simulink model "LCK_AVP"  (R2018b)
settings: Solver=FixedStepDiscrete  StartTime=0.0  StopTime=inf  FixedStep=0.01  RelTol=1e-3
PreLoadFcn:
  | if exist('tl_preloadfcn','file'), tl_preloadfcn(gcs,'4.4.0.41'); end
PostLoadFcn:
  | if any(exist('dsrtsu_mdlpostloadfcn', 'file') ~= 0), dsrtsu_mdlpostloadfcn('Execute', bdroot); end
  | if exist('tl_postloadfcn','file'), tl_postloadfcn(gcs,'4.4.0.41'); end
InitFcn:
  | if exist('tlds_init','file'), tlds_init(gcs); end
StartFcn:
  | if exist('tlds_start','file'), tlds_start(gcs); end
StopFcn:
  | if exist('tlds_stop','file'), tlds_stop(gcs); end
values from neighbouring files (symbols this model uses):
  C_DEG2RAD = 0.0175    [LCK_Macro.sldd]
  C_KPH2MPS = 0.2778    [LCK_Macro.sldd]
  C_NEARZERO = 0.0001    [LCK_Macro.sldd]
  C_ONE = 1.0    [LCK_Macro.sldd]
  C_RAD2DEG = 57.2958    [LCK_Macro.sldd]
  C_ZERO = 0.0    [LCK_Macro.sldd]
  k_accel_pedal_pos_per_speed_x : value not decoded    [LCK_LogicPara.sldd]
  k_accel_pedal_pos_per_speed_z : value not decoded    [LCK_LogicPara.sldd]
  k_brake_suprress_hold = 1000.0    [LCK_LogicPara.sldd]
  k_driver_appl_torque_filt = 50.0    [LCK_LogicPara.sldd]
  k_driver_suppression_hold_time = 3000.0    [LCK_LogicPara.sldd]
  k_hands_on_wheel_hold_msec = 500.0    [LCK_LogicPara.sldd]
  k_hands_on_wheel_torque_hi = 0.2    [LCK_LogicPara.sldd]
  k_hands_on_wheel_torque_lo = 0.15    [LCK_LogicPara.sldd]
  k_handsoff_delay_cycles = 50.0    [LCK_LogicPara.sldd]
  k_handsoff_torq_Lo_CR = 0.3    [LCK_LogicPara.sldd]
  k_handson_delay_cycles = 5.0    [LCK_LogicPara.sldd]
  k_HighAccel_suppress_hold = 3000.0    [LCK_LogicPara.sldd]
  k_HLR_suprress_hold = 3000.0    [LCK_LogicPara.sldd]
  k_hs_StrAng_CR_threshold_z : value not decoded    [LCK_LogicPara.sldd]
  k_LC_Exit_Switch = 0.0    [LCK_LogicPara.sldd]
  k_LCG_Configured = 1.0    [LCK_LogicPara.sldd]
  k_LCK_A0_Rdy2Act_UseConst = 0.0    [LCK_LogicPara.sldd]
  k_LCK_A0Fac_ActSta : value not decoded    [LCK_CtrlPara.sldd]
  k_LCK_A0Fac_DrvStm : value not decoded    [LCK_CtrlPara.sldd]
  k_LCK_A0Shift_LftCurv : value not decoded    [LCK_CtrlPara.sldd]
  k_LCK_A0Shift_RgtCurv : value not decoded    [LCK_CtrlPara.sldd]
  k_LCK_A0Shift_StraLan = 0.0    [LCK_CtrlPara.sldd]
  k_LCK_A0ShiftFac_Dy_LftCurv : value not decoded    [LCK_CtrlPara.sldd]
  k_LCK_A0ShiftFac_Dy_RgtCurv : value not decoded    [LCK_CtrlPara.sldd]
  k_LCK_A0ShiftFac_Vspd : value not decoded    [LCK_CtrlPara.sldd]
  k_LCK_accel_inhibit_thold = 35.0    [LCK_LogicPara.sldd]
  k_LCK_Active2Ready_Mask = 255.0    [LCK_LogicPara.sldd]
  k_LCK_CvatRateBks : value not decoded    [LCK_CtrlPara.sldd]
  k_LCK_CvatrBks : value not decoded    [LCK_CtrlPara.sldd]
  k_LCK_DFac_Dy : value not decoded    [LCK_CtrlPara.sldd]
  k_LCK_DFac_Dy_Curv : value not decoded    [LCK_CtrlPara.sldd]
  k_LCK_DFac_HaCurCen : value not decoded    [LCK_CtrlPara.sldd]
  k_LCK_DFac_HaCurSid : value not decoded    [LCK_CtrlPara.sldd]
  k_LCK_DFac_HadCurCen : value not decoded    [LCK_CtrlPara.sldd]
  k_LCK_DFac_HadCurSid : value not decoded    [LCK_CtrlPara.sldd]
  k_LCK_DFac_HadStrCen : value not decoded    [LCK_CtrlPara.sldd]
  k_LCK_DFac_HadStrSid : value not decoded    [LCK_CtrlPara.sldd]
  k_LCK_DFac_HaStrCen : value not decoded    [LCK_CtrlPara.sldd]
  k_LCK_DFac_HaStrSid : value not decoded    [LCK_CtrlPara.sldd]
  k_LCK_DFac_Rad : value not decoded    [LCK_CtrlPara.sldd]
  k_LCK_DFac_SA_CurCen : value not decoded    [LCK_CtrlPara.sldd]
  k_LCK_DFac_SA_CurSid : value not decoded    [LCK_CtrlPara.sldd]
  k_LCK_DFac_SA_StrCen : value not decoded    [LCK_CtrlPara.sldd]
  k_LCK_DFac_SA_StrSid : value not decoded    [LCK_CtrlPara.sldd]
  k_LCK_DFac_SS_CurCen : value not decoded    [LCK_CtrlPara.sldd]
  k_LCK_DFac_SS_CurSid : value not decoded    [LCK_CtrlPara.sldd]
  k_LCK_DFac_SS_StrCen : value not decoded    [LCK_CtrlPara.sldd]
  k_LCK_DFac_SS_StrSid : value not decoded    [LCK_CtrlPara.sldd]
  k_LCK_DFac_Vspd : value not decoded    [LCK_CtrlPara.sldd]
  k_LCK_DlyTm_DrvStim = 0.2    [LCK_CtrlPara.sldd]
  k_LCK_DTermMax = 2.0    [LCK_CtrlPara.sldd]
  k_LCK_DyBks_Curv : value not decoded    [LCK_CtrlPara.sldd]
  k_LCK_Enable_POOnly = 1.0    [LCK_LogicPara.sldd]
  k_LCK_Entry_DistBuffer = 0.1    [LCK_LogicPara.sldd]
  k_LCK_Fac_Vspd2RngThr_FalRec = 0.23    [LCK_CtrlPara.sldd]
  k_LCK_Ffw_CvatSwh = 0.0    [LCK_CtrlPara.sldd]
  k_LCK_Ffw_DyBks : value not decoded    [LCK_CtrlPara.sldd]
  k_LCK_Ffw_TimCon_CmdFlt = 0.0    [LCK_CtrlPara.sldd]
  k_LCK_FfwDeltaFac_Rad_Lft : value not decoded    [LCK_CtrlPara.sldd]
  k_LCK_FfwDeltaFac_Rad_Rgt : value not decoded    [LCK_CtrlPara.sldd]
  k_LCK_FfwDeltaFac_Vspd : value not decoded    [LCK_CtrlPara.sldd]
  k_LCK_FfwFac_CvatRate_Lft : value not decoded    [LCK_CtrlPara.sldd]
  k_LCK_FfwFac_CvatRate_Rgt : value not decoded    [LCK_CtrlPara.sldd]
  k_LCK_FfwFac_Dy : value not decoded    [LCK_CtrlPara.sldd]
  k_LCK_FfwFac_Rad_Lft : value not decoded    [LCK_CtrlPara.sldd]
  k_LCK_FfwFac_Rad_Rgt : value not decoded    [LCK_CtrlPara.sldd]
  k_LCK_FfwFac_Vspd : value not decoded    [LCK_CtrlPara.sldd]
  k_LCK_FfwTorq_Cvat : value not decoded    [LCK_CtrlPara.sldd]
  k_LCK_HAFac_ActSta : value not decoded    [LCK_CtrlPara.sldd]
  k_LCK_HAFac_DrvStm : value not decoded    [LCK_CtrlPara.sldd]
  k_LCK_HaloTime = 2000.0    [LCK_LogicPara.sldd]
  k_LCK_HaloTime_Switch = 0.0    [LCK_LogicPara.sldd]
  k_LCK_HARFac_ActSta : value not decoded    [LCK_CtrlPara.sldd]
  k_LCK_HARFac_DrvStm : value not decoded    [LCK_CtrlPara.sldd]
  k_LCK_Hed_DyBks : value not decoded    [LCK_CtrlPara.sldd]
  k_LCK_HedAngDiffX : value not decoded    [LCK_CtrlPara.sldd]
  k_LCK_HedAngRateDiffX : value not decoded    [LCK_CtrlPara.sldd]
  k_LCK_HndsOnWhel_DlyTm_Idl2Rdy = 0.0    [LCK_LogicPara.sldd]
  k_LCK_host_veh_width = 1.86    [LCK_LogicPara.sldd]
  k_LCK_Idle2Ready_Mask = 239.0    [LCK_LogicPara.sldd]
  k_LCK_Junc_SusTime = 1.0    [LCK_LogicPara.sldd]
  k_LCK_KpKdDecSlopeLmt = 10.0    [LCK_CtrlPara.sldd]
  k_LCK_KpKdIncSlopeLmt = 5.0    [LCK_CtrlPara.sldd]
  k_LCK_Lat_Ctrl_DFac_Lft = 1.0    [LCK_CtrlPara.sldd]
  k_LCK_Lat_Ctrl_DFac_Rgt = 1.05    [LCK_CtrlPara.sldd]
  k_LCK_Lat_Ctrl_Kd = 0.8    [LCK_CtrlPara.sldd]
  k_LCK_Lat_Ctrl_Ki = 0.5    [LCK_CtrlPara.sldd]
  k_LCK_Lat_Ctrl_Kp = 0.7    [LCK_CtrlPara.sldd]
  k_LCK_Lat_Ctrl_Kp_NearGain = 0.7    [LCK_CtrlPara.sldd]
  k_LCK_Lat_Ctrl_PFac_Lft = 1.0    [LCK_CtrlPara.sldd]
  k_LCK_Lat_Ctrl_PFac_Rgt = 1.05    [LCK_CtrlPara.sldd]
  k_LCK_Lat_Ctrl_TimCon_CmdFlt = 5.0    [LCK_CtrlPara.sldd]
  k_LCK_Lat_DFac_Rad : value not decoded    [LCK_CtrlPara.sldd]
  k_LCK_Lat_DFac_SS_Cur : value not decoded    [LCK_CtrlPara.sldd]
  k_LCK_Lat_DFac_SS_Str : value not decoded    [LCK_CtrlPara.sldd]
  k_LCK_Lat_DFac_Vspd : value not decoded    [LCK_CtrlPara.sldd]
  k_LCK_Lat_DyBks : value not decoded    [LCK_CtrlPara.sldd]
  k_LCK_Lat_IFac_Rad : value not decoded    [LCK_CtrlPara.sldd]
  k_LCK_Lat_IFac_Vspd : value not decoded    [LCK_CtrlPara.sldd]
  k_LCK_Lat_ILmtFac_Dy_CurvLan : value not decoded    [LCK_CtrlPara.sldd]
  k_LCK_Lat_ILmtFac_Dy_StraLan : value not decoded    [LCK_CtrlPara.sldd]
  k_LCK_Lat_ILmtFac_Rad : value not decoded    [LCK_CtrlPara.sldd]
  k_LCK_Lat_ILmtFac_Rad_NearGain = 1.0    [LCK_CtrlPara.sldd]
  k_LCK_Lat_ILmtFac_Vspd_CurvLan : value not decoded    [LCK_CtrlPara.sldd]
  k_LCK_Lat_ILmtFac_Vspd_StraLan : value not decoded    [LCK_CtrlPara.sldd]
  k_LCK_Lat_ITermLmt_Dy = 1.0    [LCK_CtrlPara.sldd]
  k_LCK_Lat_KpKdDecSlopeLmt = 10.0    [LCK_CtrlPara.sldd]
  k_LCK_Lat_KpKdIncSlopeLmt = 10.0    [LCK_CtrlPara.sldd]
  k_LCK_Lat_PFac_Dy_InnLftCur : value not decoded    [LCK_CtrlPara.sldd]
  k_LCK_Lat_PFac_Dy_InnRgtCur : value not decoded    [LCK_CtrlPara.sldd]
  k_LCK_Lat_PFac_Dy_OutLftCur : value not decoded    [LCK_CtrlPara.sldd]
  k_LCK_Lat_PFac_Dy_OutRgtCur : value not decoded    [LCK_CtrlPara.sldd]
  k_LCK_Lat_PFac_Dy_Str : value not decoded    [LCK_CtrlPara.sldd]
  k_LCK_Lat_PFac_Rad : value not decoded    [LCK_CtrlPara.sldd]
  ... (+153 more)
undefined symbols (not defined in the file or in its folder): k_LCK_CurvBks, K_LCK_SPA0A1A2_LMRngCmp_y
libraries: LateralControl_fcns_lib x58, simulink x24
(part 11 of 48)

== system LCK_AVP/Lateral_Control_Module/Adas_Lateral_Control_LCK_Core/Module 9 ==
  Vspd : Inport
  Dy_0 : Inport  Port=2
  Hed_Ang : Inport  Port=3
  Hed_Ang_Rat : Inport  Port=4
  Steer_Ang : Inport  Port=5
  Steer_Spd : Inport  Port=6
  Road_Radius : Inport  Port=7
  Str_Flag : Inport  Port=8
  Cen_Flag : Inport  Port=9
  Bus Creator : BusCreator  Inputs=5
  Module 0 : Subsystem
  Module 1 : Subsystem
  LatCtrl_Info : Outport
  wires:
  Dy_0/1 -> Module 0/3(Dy_0)
  Hed_Ang/1 -> Module 0/1(Hed_Ang), Module 1/1(Hed_Ang)
  Str_Flag/1 -> Module 0/4(Str_Flag)
  Vspd/1 -> Module 0/5(Vspd)
  Road_Radius/1 -> Module 0/6(Road_Radius)
  Steer_Spd/1 -> Module 0/8(Steer_Spd)
  Hed_Ang_Rat/1 -> Module 1/2(Hed_Ang_Rat), Module 0/2(Hed_Ang_Diff_Rat)
  Module 1/1(LatCtrl_Cmd) -> Bus Creator/1  "LatCtrl_Cmd"
  Cen_Flag/1 -> Module 0/9(Cen_Flag)
  Bus Creator/1 -> LatCtrl_Info/1
  Steer_Ang/1 -> Module 0/7(Steer_Ang)
  Module 0/1(P_Gain) -> Bus Creator/4, Module 1/3(P_Gain)  "LatCtrl_P"
  Module 0/2(D_Gain) -> Bus Creator/5, Module 1/4(D_Gain)  "LatCtrl_D"
  Module 1/2(LatCtrl_P_Term) -> Bus Creator/2  "LatCtrl_PTerm"
  Module 1/3(LatCtrl_D_Term) -> Bus Creator/3  "LatCtrl_DTerm"

== system LCK_AVP/Lateral_Control_Module/Adas_Lateral_Control_LCK_Core/Process of SPP False Recognition ==
  LatCtrl_LCK_LanSigInputs : Inport
  LatCtrl_LCK_TrackSigInputs : Inport  Description=_GWMAB30P4.LCK.000_220_  Port=2
  Vspd : Inport  Port=3
  Bus Selector20 : BusSelector  OutputSignals=CIPV1ObjRange,CIPV1ObjTrackID
  Bus Selector21 : BusSelector  OutputSignals=VID_Lin_01_Range,VID_Lin_02_Range
  Constant10 : Constant  Value=0  OutDataTypeStr=uint8
  Constant2 : Constant  Value=4  OutDataTypeStr=uint8
  Constant5 : Constant  Value=0  OutDataTypeStr=uint8
  Constant6 : Constant  Value=2  OutDataTypeStr=uint8
  Constant8 : Constant  Value=2  OutDataTypeStr=uint8
  Constant9 : Constant  Value=3  OutDataTypeStr=uint8
  Divide1 : Product  Description=_GWMAB30P3.LCK.000_157_  Inputs=*/  OutDataTypeStr=single
  Product6 : Product
  Relational Operator : RelationalOperator  OutDataTypeStr=boolean  RndMeth=Nearest
  Relational Operator1 : RelationalOperator  Operator=>  OutDataTypeStr=boolean  RndMeth=Nearest
  Relational Operator2 : RelationalOperator  Operator=<  OutDataTypeStr=boolean  RndMeth=Nearest
  Sum3 : Sum  Description=_GWMAB30P2.LCK.000_1362_
  Switch1 : Switch  Description=_GWMAB30P2.LCK.000_1368_  Threshold=0.5  OutDataTypeStr=uint8
  Switch10 : Switch  Description=_GWMAB30P2.LCK.000_1368_  Threshold=0.5
  Switch8 : Switch  Description=_GWMAB30P2.LCK.000_1368_  Threshold=0.5  OutDataTypeStr=uint8
  k_LCK_Fac_Vspd2RngThr_FalRec : Constant  Value=k_LCK_Fac_Vspd2RngThr_FalRec
  k_LCK_RngThr_FalRec : Lookup_n-D  NumberOfTableDimensions=1  BreakpointsForDimension1=k_LCK_VspdBks  Table=k_LCK_RngThr_FalRec  ExtrapMethod=Clip  InternalRulePriority=Speed  RndMeth=Simplest  InputSameDT=on
  SPP_Recognition_Type : Outport
  wires:
  LatCtrl_LCK_LanSigInputs/1 -> Bus Selector21/1
  LatCtrl_LCK_TrackSigInputs/1 -> Bus Selector20/1
  Constant5/1 -> Relational Operator1/2
  Relational Operator2/1 -> Switch10/2
  k_LCK_Fac_Vspd2RngThr_FalRec/1 -> Product6/1
  Constant9/1 -> Switch10/3
  Constant10/1 -> Switch8/3
  Switch8/1 -> SPP_Recognition_Type/1
  Constant6/1 -> Divide1/2
  Constant8/1 -> Switch10/1
  Relational Operator/1 -> Switch8/2
  Relational Operator1/1 -> Switch1/2
  Constant2/1 -> Switch1/3
  Switch10/1 -> Switch1/1
  Switch1/1 -> Switch8/1
  Bus Selector20/2 -> Relational Operator1/1  "<CIPV1ObjTrackID>"
  Product6/1 -> Relational Operator2/1
  Bus Selector20/1 -> Relational Operator2/2  "<CIPV1ObjRange>"
  Vspd/1 -> Product6/2, k_LCK_RngThr_FalRec/1
  k_LCK_RngThr_FalRec/1 -> Relational Operator/1
  Bus Selector21/1 -> Sum3/1  "<VID_Lin_01_Range>"
  Bus Selector21/2 -> Sum3/2  "<VID_Lin_02_Range>"
  Sum3/1 -> Divide1/1
  Divide1/1 -> Relational Operator/2

== system LCK_AVP/Lateral_Control_Module/LCK_State_Ctrl/Det_Driver_Operation ==
  veh_speed_kph : Inport  Description=_GWMAB30P4.LCK.000_82_
  TorsionBarTorque : Inport  Description=_GWMH9P3.Latctrl.000_23_  Port=2
  Steer_Angle_iso : Inport  Description=_GWMH9P3.Latctrl.000_23_  Port=3
  BrkPedalApp : Inport  Description=_GWMH9P3.Latctrl.000_23_  Port=4
  AccPedalPosition : Inport  Description=_GWMH9P3.Latctrl.000_23_  Port=5
  Gear_Pos : Inport  Description=_GWMH9P3.Latctrl.000_23_  Port=6
  steer_angle_CR_iso : Inport  Description=_GWMH9P3.Latctrl.000_23_  Port=7
  DirectionIndSwitchPos : Inport  Description=_GACA26P3.Latctrl.000_20_  Port=8
  LCK_Mode : Inport  Port=9
  Final_Torq_Cmd : Inport  Port=10
  Det_Driver_Steer_Override : Subsystem  Description=_GWMAB30P4.Latctrl.000_122_  TreatAsAtomicUnit=on
  Det_Driver_Suppression : Subsystem
  Det_Hands_on_Wheel : Subsystem
  Filter_Accel_Pedal : Subsystem  Description=_GWMAB30P4.Latctrl.000_101_  TreatAsAtomicUnit=on
  Filter_steer_angle_CR : Subsystem  Description=_GWMAB30P4.Latctrl.000_122_  TreatAsAtomicUnit=on
  f_hands_on_wheel : Outport
  f_driver_override_left_trq : Outport  Port=2
  f_driver_override_right_trq : Outport  Port=3
  f_Left_driver_suppression : Outport  Port=4
  f_Right_driver_suppression : Outport  Port=5
  wires:
  Steer_Angle_iso/1 -> [steer_angle_iso], Det_Driver_Suppression/1(steer_angle_iso)
  veh_speed_kph/1 -> [Vspd], Filter_Accel_Pedal/3(IP_vehicle_speed)
  [Vspd] -> Filter_steer_angle_CR/3(IP_veh_spd_kph)
  [steer_angle_iso] -> Filter_steer_angle_CR/1(steer_angle_iso)
  steer_angle_CR_iso/1 -> Filter_steer_angle_CR/2(steer_angle_CR_iso)
  Gear_Pos/1 -> Filter_Accel_Pedal/2(GearLeverPos)
  [Vspd] -> Det_Driver_Steer_Override/3(Vspd)
  Filter_Accel_Pedal/1(f_LCK_accel_pedal_inhibit) -> Det_Driver_Suppression/3(f_LCK_steering_angle_CR_inhibit)
  AccPedalPosition/1 -> Filter_Accel_Pedal/1(Accel_Pedal_Posn)
  TorsionBarTorque/1 -> [TorsionBarTorque], Det_Hands_on_Wheel/1(TorsionBarTorque)
  Filter_steer_angle_CR/1(f_LCK_steering_angle_CR_inhibit) -> Det_Driver_Suppression/4(f_LCK_accel_pedal_inhibit)
  BrkPedalApp/1 -> Det_Driver_Suppression/2(f_brake_pedal_inhibit)
  LCK_Mode/1 -> Det_Driver_Steer_Override/1(LCK_Mode)
  Det_Driver_Steer_Override/1(f_driver_override_left_trq) -> f_driver_override_left_trq/1
  Final_Torq_Cmd/1 -> Det_Driver_Steer_Override/2(Final_Torq_Cmd)
  [TorsionBarTorque] -> Det_Driver_Steer_Override/4(Steer_Torq)
  Det_Driver_Suppression/2(f_Right_driver_suppression) -> f_Right_driver_suppression/1
  Det_Driver_Suppression/1(f_Left_driver_suppression) -> f_Left_driver_suppression/1
  Det_Driver_Steer_Override/2(f_driver_override_right_trq) -> f_driver_override_right_trq/1
  Det_Hands_on_Wheel/1(f_hands_on_wheel) -> f_hands_on_wheel/1
  DirectionIndSwitchPos/1 -> Det_Driver_Suppression/5(DirectionIndSwitchPos)
